simulink model "Planta_con_resorte"  (R2020a)
settings: Solver=VariableStepAuto  StartTime=0.0  StopTime=10.0  RelTol=1e-3
undefined symbols (not defined in the file): bm, K_motor, k_resorte, L, m_total, R
settings Model: Creator=Adriana  LastModifiedBy=Noxi-PC

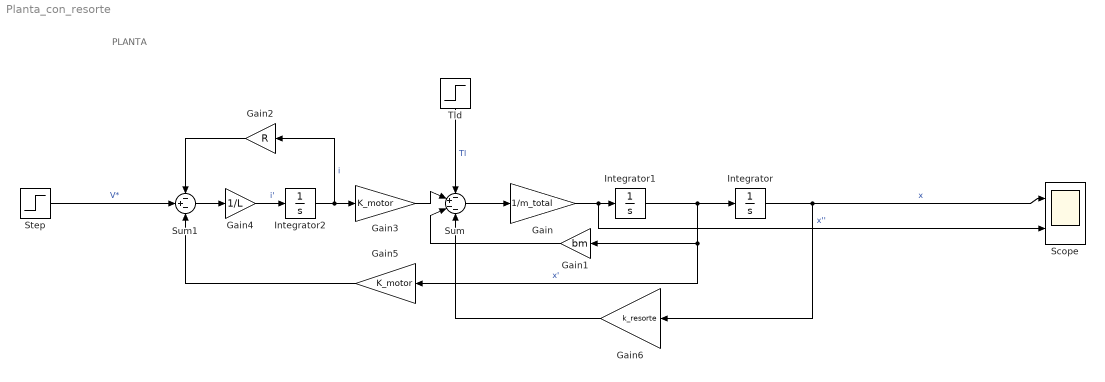
== system Planta_con_resorte ==
  note: PLANTA
  Gain : Gain  Gain=1/m_total
  Gain1 : Gain  Gain=bm
  Gain2 : Gain  Gain=R
  Gain3 : Gain  Gain=K_motor
  Gain4 : Gain  Gain=1/L
  Gain5 : Gain  Gain=K_motor
  Gain6 : Gain  Gain=k_resorte
  Integrator : Integrator
  Integrator1 : Integrator
  Integrator2 : Integrator
  Scope : Scope  NumInputPorts=2
  Step : Step  After=0  SampleTime=0
  Sum : Sum  Inputs=-+--
  Sum1 : Sum  Inputs=-+-
  Tld : Step  Time=2  SampleTime=0
  wires:
  Integrator1/1 -> Gain5/1, Gain1/1, Integrator/1  "x'"
  Integrator/1 -> Scope/1, Gain6/1  "x"
  Gain/1 -> Scope/2, Integrator1/1  "x''"
  Sum/1 -> Gain/1
  Gain1/1 -> Sum/3
  Tld/1 -> Sum/1  "Tl"
  Gain3/1 -> Sum/2
  Integrator2/1 -> Gain2/1, Gain3/1  "i"
  Sum1/1 -> Gain4/1
  Gain4/1 -> Integrator2/1  "i'"
  Gain2/1 -> Sum1/1
  Gain5/1 -> Sum1/3
  Step/1 -> Sum1/2  "V*"
  Gain6/1 -> Sum/4
